simulink model "simuUnaValvula"  (R2018a)
settings: Solver=VariableStepAuto  StartTime=0.0  StopTime=inf  RelTol=1e-3
libraries: simulink x1, pePwmGenerator x1, vrlib x1
settings Model: Creator=Ruben  LastModifiedBy=Ruben

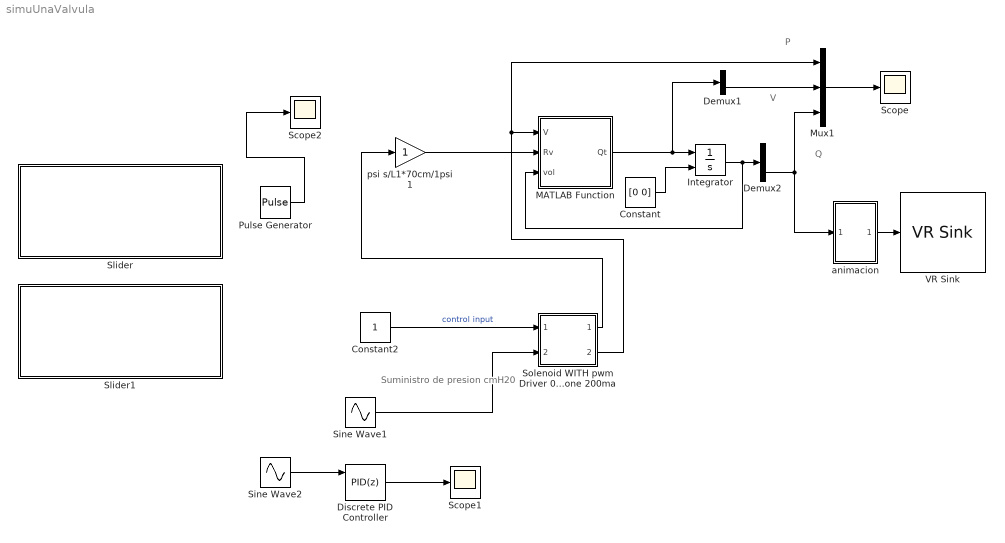
== system simuUnaValvula ==
  note: Suministro de presion
      | cmH20
  note: Q
  note: P
  note: V
  Constant : Constant  Value="[0    0]"
  Constant2 : Constant
  Demux1 : Demux  Outputs=2
  Demux2 : Demux  Outputs=2
  Discrete PID Controller : simulink/Continuous/PID Controller  Controller=PID  TimeDomain=Discrete-time  SampleTime=.1  IntegratorMethod=Forward Euler  FilterMethod=Forward Euler  Form=Parallel  UseFilter=on  ControllerParametersSource=internal  P=1  I=1  D=0  N=100  InitialConditionSource=internal  InitialConditionForIntegrator=0  InitialConditionForFilter=0  ExternalReset=rising  LimitOutput=off  UpperSaturationLimit=inf  LowerSaturationLimit=-inf  LinearizeAsGain=off  AntiWindupMode=none  Kb=1  TrackingMode=off  Kt=1  PParamMin=[]  PParamMax=[]  IParamMin=[]  IParamMax=[]  DParamMin=[]  DParamMax=[]  NParamMin=[]  NParamMax=[]  KbParamMin=[]  KbParamMax=[]  KtParamMin=[]  KtParamMax=[]  POutMin=[]  POutMax=[]  IOutMin=[]  IOutMax=[]  DOutMin=[]  DOutMax=[]  NOutMin=[]  NOutMax=[]  KbOutMin=[]  KbOutMax=[]  KtOutMin=[]  KtOutMax=[]  IntegratorOutMin=[]  IntegratorOutMax=[]  FilterOutMin=[]  FilterOutMax=[]  SumOutMin=[]  SumOutMax=[]  SumI1OutMin=[]  SumI1OutMax=[]  SumI2OutMin=[]  SumI2OutMax=[]  SumI3OutMin=[]  SumI3OutMax=[]  SumDOutMin=[]  SumDOutMax=[]  SaturationOutMin=[]  SaturationOutMax=[]  IntegratorContinuousStateAttributes=''  IntegratorStateMustResolveToSignalObject=off  IntegratorRTWStateStorageClass=Auto  FilterContinuousStateAttributes=''  FilterStateMustResolveToSignalObject=off  FilterRTWStateStorageClass=Auto  DifferentiatorICPrevScaledInput=0  DifferentiatorOutMin=[]  DifferentiatorOutMax=[]  FilterDiffOutCoefMin=[]  FilterDiffOutCoefMax=[]  SumDenOutMin=[]  SumDenOutMax=[]  SumNumOutMin=[]  SumNumOutMax=[]  ReciprocalOutMin=[]  ReciprocalOutMax=[]  DivideOutMin=[]  DivideOutMax=[]  TunerSelectOption=Transfer Function Based (PID Tuner App)
  Integrator : Integrator  InitialConditionSource=external
  MATLAB Function : MATLAB Function  TreatAsAtomicUnit=on
  Mux1 : Mux  Inputs=3
  Pulse Generator : DiscretePulseGenerator  PulseType=Time based  Period=0.4695652173913  PulseWidth=20
  Scope : Scope
  Scope1 : Scope
  Scope2 : Scope
  Sine Wave1 : Sin  Amplitude=2.5  Frequency=1.57  SampleTime=0
  Sine Wave2 : Sin  Amplitude=2.5  Frequency=1.57  SampleTime=0
  Slider : Subsystem  DialogController=hmiCreateDDGDialog  IsWebBlock=on  mask(MWDashboardBlock){webBlockId=5c75009d-8c8d-43fb-88f0-46defad8d923, webBlockType=slider, ShowInLibBrowser=on, ShowInitialText=on, HMISrcModelName=simuUnaValvula}
      mask prompts: webBlockId "WebBlock Id"; webBlockType "WebBlock Type"; HMISrcModelName "Source Model"
      mask help: SimulinkHMI:dialogs:SliderDialogDesc
      mask Help: helpview([docroot '/mapfiles/simulink.map'], 'hmi_slider')
      mask Display:
      | if strcmp(get_param(bdroot(gcb),'BlockDiagramType'), 'library')
      |     image([(matlabroot) '/toolbox/simulink/hmi/icons/Slider.png']);
      | end
  Slider1 : Subsystem  DialogController=hmiCreateDDGDialog  IsWebBlock=on  mask(MWDashboardBlock){webBlockId=99f10f40-54f3-4e18-818e-e2eb05ba8e4b, webBlockType=slider, ShowInLibBrowser=on, ShowInitialText=on, HMISrcModelName=simuUnaValvula}
      mask prompts: webBlockId "WebBlock Id"; webBlockType "WebBlock Type"; HMISrcModelName "Source Model"
      mask help: SimulinkHMI:dialogs:SliderDialogDesc
      mask Help: helpview([docroot '/mapfiles/simulink.map'], 'hmi_slider')
      mask Display:
      | if strcmp(get_param(bdroot(gcb),'BlockDiagramType'), 'library')
      |     image([(matlabroot) '/toolbox/simulink/hmi/icons/Slider.png']);
      | end
  Solenoid WITH pwm Driver 0v  closed to 1v fully  open min Resi=0.366 at 600ma (1 volt) dead zone 200ma : Subsystem  TreatAsAtomicUnit=on
      mask Display: image('C:\Users\Ruben\Downloads\Proportional-Safety_Valve.jpg');
  VR Sink : vrlib/VR Sink  InstantiateOnLoad=on  SampleTime=0.1  ViewEnable=on  RemoteChange=off  RemoteView=off  FieldsWritten=lungs.scale.3.1.1.double  WorldFileName=Lungs2.wrl  AutoView=off  VideoDimensions=[]  AllowVariableSize=off  mask(Virtual Reality Sink){}
      settings: SourceProductBaseCode=VR
      mask Display: image('C:\Users\Ruben\Downloads\animacion.png');
  animacion : Subsystem  TreatAsAtomicUnit=on
  psi s/L1*70cm/1psi 1 : Gain
  wires:
  MATLAB Function/1(Qt) -> Demux1/1, Integrator/1
  Integrator/1 -> Demux2/1, MATLAB Function/3(vol)
  Constant/1 -> Integrator/2
  Constant2/1 -> Solenoid WITH pwm Driver 0v  closed to 1v fully  open min Resi=0.366 at 600ma (1 volt) dead zone 200ma/1("Volts ")  "control input"
  Solenoid WITH pwm Driver 0v  closed to 1v fully  open min Resi=0.366 at 600ma (1 volt) dead zone 200ma/1(Req(PSI.min/L)ma) -> psi s/L1*70cm/1psi 1/1
  psi s/L1*70cm/1psi 1/1 -> MATLAB Function/2(Rv)
  Sine Wave1/1 -> Solenoid WITH pwm Driver 0v  closed to 1v fully  open min Resi=0.366 at 600ma (1 volt) dead zone 200ma/2(Pesion)
  Demux2/2 -> animacion/1(In1), Mux1/3
  Mux1/1 -> Scope/1
  Demux1/2 -> Mux1/2
  animacion/1(Out1) -> VR Sink/1
  Solenoid WITH pwm Driver 0v  closed to 1v fully  open min Resi=0.366 at 600ma (1 volt) dead zone 200ma/2(Presion) -> Mux1/1, MATLAB Function/1(V)
  Sine Wave2/1 -> Discrete PID Controller/1
  Discrete PID Controller/1 -> Scope1/1
  Pulse Generator/1 -> Scope2/1

== system simuUnaValvula/Slider ==

== system simuUnaValvula/Slider1 ==

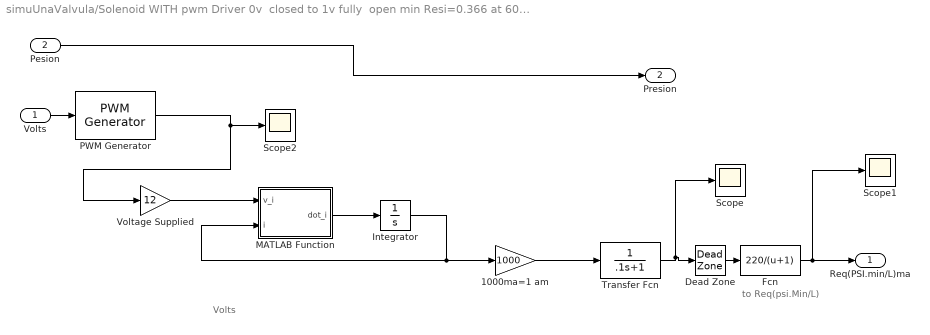
== system simuUnaValvula/Solenoid WITH pwm Driver 0v  closed to 1v fully  open min Resi=0.366 at 600ma (1 volt) dead zone 200ma ==
  note: to Req(psi.Min/L)
  note: Volts
  "Volts " : Inport
  Pesion : Inport  Port=2
  1000ma=1 am : Gain  Gain=1000
  Dead Zone : DeadZone  LowerValue=0  UpperValue=200  SaturateOnIntegerOverflow=on
  Fcn : Fcn  Expr=220/(u+1)
  Integrator : Integrator
  MATLAB Function : MATLAB Function  TreatAsAtomicUnit=on
  PWM Generator : pePwmGenerator/PWM Generator  CarrCount=Up  Tper=0.1  Ts=5e-5
  Scope : Scope
  Scope1 : Scope
  Scope2 : Scope
  Transfer Fcn : TransferFcn  Denominator=[.1 1]
  Voltage Supplied : Gain  Gain=12
  Req(PSI.min/L)ma : Outport
  Presion : Outport  Port=2
  wires:
  Integrator/1 -> 1000ma=1 am/1, MATLAB Function/2(i)
  MATLAB Function/1(dot_i) -> Integrator/1
  1000ma=1 am/1 -> Transfer Fcn/1
  Fcn/1 -> Scope1/1, Req(PSI.min/L)ma/1
  Dead Zone/1 -> Fcn/1
  Transfer Fcn/1 -> Dead Zone/1, Scope/1
  PWM Generator/1 -> Voltage Supplied/1, Scope2/1
  "Volts "/1 -> PWM Generator/1
  Voltage Supplied/1 -> MATLAB Function/1(v_i)
  Pesion/1 -> Presion/1

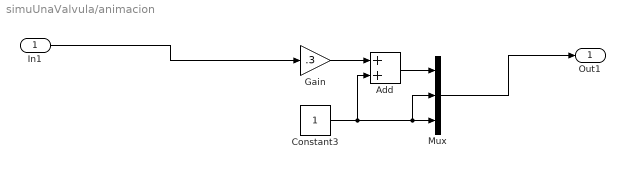
== system simuUnaValvula/animacion ==
  In1 : Inport
  Add : Sum
  Constant3 : Constant
  Gain : Gain  Gain=.3
  Mux : Mux  Inputs=3
  Out1 : Outport
  wires:
  Constant3/1 -> Add/2, Mux/2, Mux/3
  In1/1 -> Gain/1
  Add/1 -> Mux/1
  Gain/1 -> Add/1
  Mux/1 -> Out1/1

== matlab function simuUnaValvula/Solenoid WITH pwm Driver 0v  closed to 1v fully  open min Resi=0.366 at 600ma (1 volt) dead zone 200ma/MATLAB Function ==
  data: v_i input; dot_i output; i input
function dot_i = fcn(v_i,i)
R=15; % R igual a 2 ohm
%L=.063 ;% L aprox 63mh
L=.063;
dot_i = (1/L)*(v_i-R*i);

== matlab function simuUnaValvula/MATLAB Function ==
  data: V input; Rv input; Qt output; vol input
function Qt  = fcn(V,Rv,vol)
intI2=vol(1);
intI3=vol(2);
Rc=1;Rp=1; %R1=RC,R2=Rp
Cs=.005;Cl=0.2; Cw=0.2;%C1=Cs; C2=Cl*CW
%Q=I3,Qa=I2



%C2=Cl+Cw
Q=(1/(Rc+Rv))*(V-(1/Cs)*(-intI2+intI3));
Qa=(1/Rp)*(V-Q*(Rc+Rv)-(1/(Cl+Cw))*intI2);

Qt = [ Qa  Q];
